simulink model "dspace_2019"  (R2019b)
settings: Solver=FixedStepDiscrete  StartTime=0.0  StopTime=Inf  FixedStep=1e-3  RelTol=1e-3
PostLoadFcn:
  | , if any(exist('dsrtsu_mdlpostloadfcn', 'file') ~= 0), dsrtsu_mdlpostloadfcn('Execute', bdroot); end,
undefined symbols (not defined in the file): ami, amk1_setpoints_1, amk2_setpoints_1, amk3_setpoints_1, amk4_setpoints_1, as, digital, ebs, indicator, mcu_set_dbu_indicator_points, mcu_set_ecu_indicator_points, res_ntm_node_control
libraries: rtican x63, simulink x5, rti1401lib_dio_type3 x4, simulink_extras x1
(part 11 of 16)

== system dspace_2019/CAN RX/ebs_status ==
  clock_time : Clock
  ebs_status1 : rtican/RTICAN Receive (RX)   Reserved1=[]  Reserved2=[]  Reserved3=[]  Reserved4=[]  SfcnMessage=[]  Msg_Struct=[]  BoardTypeNo=[]  BoardNo=[]  ChannelNo=[]  Parameters=[]  DialogFcn=[]  UnitName=[]  Revision=[]  UnitValues=[]  DSProperties=struct('RTI',struct('Version',uint32(5),'BlockType',struct('isSLSource',uint8(1),'isSLSink',uint8(1),'isHWSource',uint8(0),'isHWSink',uint8(0),'isSetup',uint8(0),'isInline',uint8(1),'isNonInline',uint8(0),'isInterrupt',uint8(0),'isChannelwise',uint8(0)),'IOBoardType','RTICAN','UnitType','MESSAGE','Identifier','RX','DialogType','MSVC','BlockSet','RTICAN','SlaveProcessor','CAN'))  RTIBlockInterface=struct('OutputPortsWidth',int32([1 1 1 1 1 1 1]),'OutputPortsActive',[1 1 1 1 1 1 1],'OutputPortsName',{{'SC_TSMS_status','RES_open','ebs_pressure_1','ebs_pressure_2',['RX status'],['RX time'],['RX delta time']}},'OutputPortsDataType',{{'SS_DOUBLE','SS_DOUBLE','SS_DOUBLE','SS_DOUBLE','SS_DOUBLE','SS_DOUBLE','SS_DOUBLE'}},'OutputPortsLabel',{{'SC_TSMS_status','RES_open','ebs_pressure_1','ebs_pressure_2','','',''}},'OutputPortsLabelMode','ON','InputPortsWidth',int32(0),'InputPortsActive',0,'DialogFcn','rtican_message_interface_gui','BlockDisplay',{{'','center'}},'IconTransparency','on','ParameterTunableNames',{{}},'InitLevel',3,'BlockName',struct('Token',{{'ebs_status'}}),'SampleTime',{{-1}},'TriggerPort',{{'none'}},'EnablePort',{{'none'}})  RTIBlockParameters=struct('BoardTypeNo',{{1,'OFF',[]}},'BoardNo',{{1,'ON',[1 16]}},'ChannelNo',{{2,'ON',[1 2]}},'Parameters',{{struct('DataFileSupport',struct('DataFileSelectedMaster',1,'DataFileSelectedLocal',1,'DataFileName','c:\users\oscar\documents\github\sw_infrastructure\kthfspe_python\databases\can1.dbc|','DataFileDate',{{{['10-Jul-2022 16:14:04']}}},'SelectedFile','c:\users\oscar\documents\github\sw_infrastructure\kthfspe_python\databases\can1.dbc'),'Options',struct('StatusSelected',1,'TimeSelected',1,'DeltaTimeSelected',1,'BytePortSelected',0,'MessageLengthSelected',0,'TriggerPort',struct('Selected',0,'TriggerType',0),'UserCoding',struct('Selected',0,'InterfaceFile','UserDecodingFile','FcnName','UserDecodeFcn','InportSelected',0,'InportWidth',1,'OutportSelected',0,'OutportWidth',1),'EnablePortSelected',0,'SignalOnPortnameSelected',1,'UseRXService',0),'Message',struct('MsgOnBlocknameSelected',1,'MsgName','ebs_status','MsgIdFormat',0,'MsgId',80,'MsgLength',4,'NumSignals',4,'SampleTime',-1,'Signal',struct('SgnName',{'SC_TSMS_status','RES_open','ebs_pressure_1','ebs_pressure_2'},'SgnStartBit',{0,1,8,20},'SgnLength',{1,1,12,12},'SgnType',{0,0,0,0},'ModeValue',{-1,-1,-1,-1},'DataType',{0,0,0,0},'ByteLayout',{0,0,0,0},'Factor',{1,1,1,1},'Offset',{0,0,0,0},'SgnComment',{{''},{''},{''},{''}},'SgnUnit',{'','','',''},'Min',{0,0,0,0},'Max',{0,0,0,0},'SLDataType',{'SS_DOUBLE','SS_DOUBLE','SS_DOUBLE','SS_DOUBLE'}),'MsgIdNumFormat',0,'MsgComment',{{''}}),'Version',1.2,'general',struct('isFromLib',0)),'OFF',[]}},'GroupId',{{struct('Group',{{'RTICAN'}},'No',1,'Behavior',{{'NAMECHANGE'}},'BlockType',{{'SINK'}},'NameChangeFlag',0),'OFF',[]}},'SFcnRTICANMessage',{{struct('MsgType','RX','SFcnPortType','Scalar','MsgName','ebs_status','MsgIdFormat','STD','MsgId',80,'MsgLength',4,'NumSignals',4,'SampleTime',-1,'Signal',struct('SgnName',{'SC_TSMS_status','RES_open','ebs_pressure_1','ebs_pressure_2'},'SgnStartBit',{0,1,8,20},'SgnLength',{1,1,12,12},'SgnType',{'standard','standard','standard','standard'},'ModeValue',{-1,-1,-1,-1},'DataType',{['unsigned int'],['unsigned int'],['unsigned int'],['unsigned int']},'ByteLayout',{['little endian'],['little endian'],['little endian'],['little endian']},'Factor',{1,1,1,1},'Offset',{0,0,0,0},'SLDataType',{'SS_DOUBLE','SS_DOUBLE','SS_DOUBLE','SS_DOUBLE'}),'StatusSelected','yes','TimeSelected','yes','DeltaTimeSelected','yes','BytePortSelected','no','MessageLengthSelected','no','TriggerPort',struct('Selected','no','TriggerType',0),'UserCoding',struct('Selected','no','InterfaceFile','UserDecodingFile','FcnName','UserDecodeFcn','InportSelected','no','InportWidth',1,'OutportSelected','no','OutportWidth',1),'EnablePortSelected','no','UseRXService','no','BoardType','DS1','BoardNo',1,'ControllerNo',1),'OFF',[]}},'TLCFileName',{{'rtican_rx_message','OFF',[]}})  RTISFcnParameters=struct('SFcnRTICANMessage','struct','TLCFileName','char')  RTIBlockParaDefault=struct('BoardTypeNo',4302,'BoardNo',1,'ChannelNo',1,'Parameters',struct('DataFileSupport',struct('DataFileSelectedMaster',0,'DataFileSelectedLocal',0,'DataFileName','','DataFileDate','','SelectedFile',['<no file selected>']),'Options',struct('StatusSelected',1,'TimeSelected',1,'DeltaTimeSelected',1,'BytePortSelected',0,'MessageLengthSelected',0,'TriggerPort',struct('Selected',0,'TriggerType','rising'),'UserCoding',struct('Selected',0,'InterfaceFile','UserDecodingFile','FcnName','UserDecodeFcn','InportSelected',0,'InportWidth',1,'OutportSelected',0,'OutportWidth',1),'EnablePortSelected',0,'SignalOnPortnameSelected',1,'UseRXService',0),'Message',struct('MsgOnBlocknameSelected',0,'MsgName',['RX Message'],'MsgIdFormat',0,'MsgId',100,'MsgLength',8,'NumSignals',1,'SampleTime',-1,'Signal',struct('SgnName',['RX signal'],'SgnStartBit',0,'SgnLength',8,'SgnType',0,'ModeValue',-1,'DataType',0,'SLDataType','SS_DOUBLE','ByteLayout',0,'Factor',1,'Offset',0,'Min',0,'Max',255,'SgnComment',{{}},'SgnUnit',''),'MsgIdNumFormat',0,'MsgComment',{{''}}),'Version',1.2,'general',struct('isFromLib',1)),'GroupId',struct('Group',{{'RTICAN'}},'No',1,'Behavior',{{'NAMECHANGE'}},'BlockType',{{'SINK'}},'NameChangeFlag',0),'SFcnRTICANMessage',struct('MsgType','RX','MsgName',['RX Message'],'MsgIdFormat','STD','MsgId',100,'MsgLength',8,'NumSignals',1,'SampleTime',-1,'Signal',struct('SgnName',['RX signal'],'SgnStartBit',0,'SgnLength',8,'SgnType','standard','ModeValue',-1,'DataType',['unsigned int'],'ByteLayout',['little endian'],'SLDataType','SS_DOUBLE','Factor',1,'Offset',0),'StatusSelected','yes','TimeSelected','yes','DeltaTimeSelected','yes','BytePortSelected','no','MessageLengthSelected','no','EnablePortSelected','no','UserCoding',struct('Selected','no','InterfaceFile','UserDecodingFile','FcnName','UserDecodeFcn','InportSelected','no','InportWidth',1,'OutportSelected','no','OutportWidth',1),'TriggerPort',struct('Selected','no','TriggerType','rising'),'UseRXService','no','BoardType','DS4302','BoardNo',1,'ControllerNo',1,'SFcnPortType','Scalar'),'TLCFileName','rtican_rx_message')
      settings: AttributesFormatString=Group Id: RTICAN1\n  SourceProductName=dSPACE RTI CAN Blockset
  sub_time : Sum  Inputs=+-
  SC_TSMS_status_bus : Outport  PortName=signals  Element=SC_TSMS_status
  RES_open_bus : Outport  PortName=signals  Element=RES_open
  ebs_pressure_1_bus : Outport  PortName=signals  Element=ebs_pressure_1
  ebs_pressure_2_bus : Outport  PortName=signals  Element=ebs_pressure_2
  status : Outport  Port=2
  time : Outport  Port=3
  delta : Outport  Port=4
  wires:
  clock_time/1 -> sub_time/1
  sub_time/1 -> time/1
  ebs_status1/5 -> status/1
  ebs_status1/6 -> sub_time/2
  ebs_status1/7 -> delta/1
  ebs_status1/1 -> SC_TSMS_status_bus/1  "SC_TSMS_status"
  ebs_status1/2 -> RES_open_bus/1  "RES_open"
  ebs_status1/3 -> ebs_pressure_1_bus/1  "ebs_pressure_1"
  ebs_status1/4 -> ebs_pressure_2_bus/1  "ebs_pressure_2"

== system dspace_2019/CAN RX/ecu_status ==
  clock_time : Clock
  ecu_status1 : rtican/RTICAN Receive (RX)   Reserved1=[]  Reserved2=[]  Reserved3=[]  Reserved4=[]  SfcnMessage=[]  Msg_Struct=[]  BoardTypeNo=[]  BoardNo=[]  ChannelNo=[]  Parameters=[]  DialogFcn=[]  UnitName=[]  Revision=[]  UnitValues=[]  DSProperties=struct('RTI',struct('Version',uint32(5),'BlockType',struct('isSLSource',uint8(1),'isSLSink',uint8(1),'isHWSource',uint8(0),'isHWSink',uint8(0),'isSetup',uint8(0),'isInline',uint8(1),'isNonInline',uint8(0),'isInterrupt',uint8(0),'isChannelwise',uint8(0)),'IOBoardType','RTICAN','UnitType','MESSAGE','Identifier','RX','DialogType','MSVC','BlockSet','RTICAN','SlaveProcessor','CAN'))  RTIBlockInterface=struct('OutputPortsWidth',int32([1 1 1 1 1 1]),'OutputPortsActive',[1 1 1 1 1 1],'OutputPortsName',{{'rst_button','close_airs','ts_off',['RX status'],['RX time'],['RX delta time']}},'OutputPortsDataType',{{'SS_DOUBLE','SS_DOUBLE','SS_DOUBLE','SS_DOUBLE','SS_DOUBLE','SS_DOUBLE'}},'OutputPortsLabel',{{'rst_button','close_airs','ts_off','','',''}},'OutputPortsLabelMode','ON','InputPortsWidth',int32(0),'InputPortsActive',0,'DialogFcn','rtican_message_interface_gui','BlockDisplay',{{'','center'}},'IconTransparency','on','ParameterTunableNames',{{}},'InitLevel',3,'BlockName',struct('Token',{{'ecu_status'}}),'SampleTime',{{-1}},'TriggerPort',{{'none'}},'EnablePort',{{'none'}})  RTIBlockParameters=struct('BoardTypeNo',{{1,'OFF',[]}},'BoardNo',{{1,'ON',[1 16]}},'ChannelNo',{{2,'ON',[1 2]}},'Parameters',{{struct('DataFileSupport',struct('DataFileSelectedMaster',1,'DataFileSelectedLocal',1,'DataFileName','c:\users\oscar\documents\github\sw_infrastructure\kthfspe_python\databases\can1.dbc|','DataFileDate',{{{['10-Jul-2022 16:14:04']}}},'SelectedFile','c:\users\oscar\documents\github\sw_infrastructure\kthfspe_python\databases\can1.dbc'),'Options',struct('StatusSelected',1,'TimeSelected',1,'DeltaTimeSelected',1,'BytePortSelected',0,'MessageLengthSelected',0,'TriggerPort',struct('Selected',0,'TriggerType',0),'UserCoding',struct('Selected',0,'InterfaceFile','UserDecodingFile','FcnName','UserDecodeFcn','InportSelected',0,'InportWidth',1,'OutportSelected',0,'OutportWidth',1),'EnablePortSelected',0,'SignalOnPortnameSelected',1,'UseRXService',0),'Message',struct('MsgOnBlocknameSelected',1,'MsgName','ecu_status','MsgIdFormat',0,'MsgId',72,'MsgLength',8,'NumSignals',3,'SampleTime',-1,'Signal',struct('SgnName',{'rst_button','close_airs','ts_off'},'SgnStartBit',{0,8,16},'SgnLength',{8,8,8},'SgnType',{0,0,0},'ModeValue',{-1,-1,-1},'DataType',{0,0,0},'ByteLayout',{0,0,0},'Factor',{1,1,1},'Offset',{0,0,0},'SgnComment',{{''},{''},{''}},'SgnUnit',{'','',''},'Min',{0,0,0},'Max',{0,0,0},'SLDataType',{'SS_DOUBLE','SS_DOUBLE','SS_DOUBLE'}),'MsgIdNumFormat',0,'MsgComment',{{''}}),'Version',1.2,'general',struct('isFromLib',0)),'OFF',[]}},'GroupId',{{struct('Group',{{'RTICAN'}},'No',1,'Behavior',{{'NAMECHANGE'}},'BlockType',{{'SINK'}},'NameChangeFlag',0),'OFF',[]}},'SFcnRTICANMessage',{{struct('MsgType','RX','SFcnPortType','Scalar','MsgName','ecu_status','MsgIdFormat','STD','MsgId',72,'MsgLength',8,'NumSignals',3,'SampleTime',-1,'Signal',struct('SgnName',{'rst_button','close_airs','ts_off'},'SgnStartBit',{0,8,16},'SgnLength',{8,8,8},'SgnType',{'standard','standard','standard'},'ModeValue',{-1,-1,-1},'DataType',{['unsigned int'],['unsigned int'],['unsigned int']},'ByteLayout',{['little endian'],['little endian'],['little endian']},'Factor',{1,1,1},'Offset',{0,0,0},'SLDataType',{'SS_DOUBLE','SS_DOUBLE','SS_DOUBLE'}),'StatusSelected','yes','TimeSelected','yes','DeltaTimeSelected','yes','BytePortSelected','no','MessageLengthSelected','no','TriggerPort',struct('Selected','no','TriggerType',0),'UserCoding',struct('Selected','no','InterfaceFile','UserDecodingFile','FcnName','UserDecodeFcn','InportSelected','no','InportWidth',1,'OutportSelected','no','OutportWidth',1),'EnablePortSelected','no','UseRXService','no','BoardType','DS1','BoardNo',1,'ControllerNo',1),'OFF',[]}},'TLCFileName',{{'rtican_rx_message','OFF',[]}})  RTISFcnParameters=struct('SFcnRTICANMessage','struct','TLCFileName','char')  RTIBlockParaDefault=struct('BoardTypeNo',4302,'BoardNo',1,'ChannelNo',1,'Parameters',struct('DataFileSupport',struct('DataFileSelectedMaster',0,'DataFileSelectedLocal',0,'DataFileName','','DataFileDate','','SelectedFile',['<no file selected>']),'Options',struct('StatusSelected',1,'TimeSelected',1,'DeltaTimeSelected',1,'BytePortSelected',0,'MessageLengthSelected',0,'TriggerPort',struct('Selected',0,'TriggerType','rising'),'UserCoding',struct('Selected',0,'InterfaceFile','UserDecodingFile','FcnName','UserDecodeFcn','InportSelected',0,'InportWidth',1,'OutportSelected',0,'OutportWidth',1),'EnablePortSelected',0,'SignalOnPortnameSelected',1,'UseRXService',0),'Message',struct('MsgOnBlocknameSelected',0,'MsgName',['RX Message'],'MsgIdFormat',0,'MsgId',100,'MsgLength',8,'NumSignals',1,'SampleTime',-1,'Signal',struct('SgnName',['RX signal'],'SgnStartBit',0,'SgnLength',8,'SgnType',0,'ModeValue',-1,'DataType',0,'SLDataType','SS_DOUBLE','ByteLayout',0,'Factor',1,'Offset',0,'Min',0,'Max',255,'SgnComment',{{}},'SgnUnit',''),'MsgIdNumFormat',0,'MsgComment',{{''}}),'Version',1.2,'general',struct('isFromLib',1)),'GroupId',struct('Group',{{'RTICAN'}},'No',1,'Behavior',{{'NAMECHANGE'}},'BlockType',{{'SINK'}},'NameChangeFlag',0),'SFcnRTICANMessage',struct('MsgType','RX','MsgName',['RX Message'],'MsgIdFormat','STD','MsgId',100,'MsgLength',8,'NumSignals',1,'SampleTime',-1,'Signal',struct('SgnName',['RX signal'],'SgnStartBit',0,'SgnLength',8,'SgnType','standard','ModeValue',-1,'DataType',['unsigned int'],'ByteLayout',['little endian'],'SLDataType','SS_DOUBLE','Factor',1,'Offset',0),'StatusSelected','yes','TimeSelected','yes','DeltaTimeSelected','yes','BytePortSelected','no','MessageLengthSelected','no','EnablePortSelected','no','UserCoding',struct('Selected','no','InterfaceFile','UserDecodingFile','FcnName','UserDecodeFcn','InportSelected','no','InportWidth',1,'OutportSelected','no','OutportWidth',1),'TriggerPort',struct('Selected','no','TriggerType','rising'),'UseRXService','no','BoardType','DS4302','BoardNo',1,'ControllerNo',1,'SFcnPortType','Scalar'),'TLCFileName','rtican_rx_message')
      settings: AttributesFormatString=Group Id: RTICAN1\n  SourceProductName=dSPACE RTI CAN Blockset
  sub_time : Sum  Inputs=+-
  rst_button_bus : Outport  PortName=signals  Element=rst_button
  close_airs_bus : Outport  PortName=signals  Element=close_airs
  ts_off_bus : Outport  PortName=signals  Element=ts_off
  status : Outport  Port=2
  time : Outport  Port=3
  delta : Outport  Port=4
  wires:
  clock_time/1 -> sub_time/1
  sub_time/1 -> time/1
  ecu_status1/4 -> status/1
  ecu_status1/5 -> sub_time/2
  ecu_status1/6 -> delta/1
  ecu_status1/1 -> rst_button_bus/1  "rst_button"
  ecu_status1/2 -> close_airs_bus/1  "close_airs"
  ecu_status1/3 -> ts_off_bus/1  "ts_off"

== system dspace_2019/CAN RX/fault ==
  clock_time : Clock
  fault1 : rtican/RTICAN Receive (RX)   Reserved1=[]  Reserved2=[]  Reserved3=[]  Reserved4=[]  SfcnMessage=[]  Msg_Struct=[]  BoardTypeNo=[]  BoardNo=[]  ChannelNo=[]  Parameters=[]  DialogFcn=[]  UnitName=[]  Revision=[]  UnitValues=[]  DSProperties=struct('RTI',struct('Version',uint32(5),'BlockType',struct('isSLSource',uint8(1),'isSLSink',uint8(1),'isHWSource',uint8(0),'isHWSink',uint8(0),'isSetup',uint8(0),'isInline',uint8(1),'isNonInline',uint8(0),'isInterrupt',uint8(0),'isChannelwise',uint8(0)),'IOBoardType','RTICAN','UnitType','MESSAGE','Identifier','RX','DialogType','MSVC','BlockSet','RTICAN','SlaveProcessor','CAN'))  RTIBlockInterface=struct('OutputPortsWidth',int32([1 1 1 1 1 1 1 1 1 1 1 1 1 1]),'OutputPortsActive',ones(1,14),'OutputPortsName',{{'unit_id','sc_open','ts_off_watchdog_triggered','apps_discrepancy','bpps_discrepancy','brake_pressure_discrepancy','steering_angle_discrepancy','apps_out_of_range','bpps_out_of_range','brake_pressure_out_of_range','steering_angle_out_of_range',['RX status'],['RX time'],['RX delta time']}},'OutputPortsDataType',{{'SS_DOUBLE','SS_DOUBLE','SS_DOUBLE','SS_DOUBLE','SS_DOUBLE','SS_DOUBLE','SS_DOUBLE','SS_DOUBLE','SS_DOUBLE','SS_DOUBLE','SS_DOUBLE','SS_DOUBLE','SS_DOUBLE','SS_DOUBLE'}},'OutputPortsLabel',{{'unit_id','sc_open','ts_off_watchdog_triggered','apps_discrepancy','bpps_discrepancy','brake_pressure_discrepancy','steering_angle_discrepancy','apps_out_of_range','bpps_out_of_range','brake_pressure_out_of_range','steering_angle_out_of_range','','',''}},'OutputPortsLabelMode','ON','InputPortsWidth',int32(0),'InputPortsActive',0,'DialogFcn','rtican_message_interface_gui','BlockDisplay',{{'','center'}},'IconTransparency','on','ParameterTunableNames',{{}},'InitLevel',3,'BlockName',struct('Token',{{'fault'}}),'SampleTime',{{-1}},'TriggerPort',{{'none'}},'EnablePort',{{'none'}})  RTIBlockParameters=struct('BoardTypeNo',{{1,'OFF',[]}},'BoardNo',{{1,'ON',[1 16]}},'ChannelNo',{{2,'ON',[1 2]}},'Parameters',{{struct('DataFileSupport',struct('DataFileSelectedMaster',1,'DataFileSelectedLocal',1,'DataFileName','c:\users\oscar\documents\github\sw_infrastructure\kthfspe_python\databases\can1.dbc|','DataFileDate',{{{['10-Jul-2022 16:14:04']}}},'SelectedFile','c:\users\oscar\documents\github\sw_infrastructure\kthfspe_python\databases\can1.dbc'),'Options',struct('StatusSelected',1,'TimeSelected',1,'DeltaTimeSelected',1,'BytePortSelected',0,'MessageLengthSelected',0,'TriggerPort',struct('Selected',0,'TriggerType',0),'UserCoding',struct('Selected',0,'InterfaceFile','UserDecodingFile','FcnName','UserDecodeFcn','InportSelected',0,'InportWidth',1,'OutportSelected',0,'OutportWidth',1),'EnablePortSelected',0,'SignalOnPortnameSelected',1,'UseRXService',0),'Message',struct('MsgOnBlocknameSelected',1,'MsgName','fault','MsgIdFormat',0,'MsgId',255,'MsgLength',8,'NumSignals',11,'SampleTime',-1,'Signal',struct('SgnName',{'unit_id','sc_open','ts_off_watchdog_triggered','apps_discrepancy','bpps_discrepancy','brake_pressure_discrepancy','steering_angle_discrepancy','apps_out_of_range','bpps_out_of_range','brake_pressure_out_of_range','steering_angle_out_of_range'},'SgnStartBit',{0,8,8,8,9,10,11,12,13,14,15},'SgnLength',{8,1,1,1,1,1,1,1,1,1,1},'SgnType',{1,2,2,2,2,2,2,2,2,2,2},'ModeValue',{-1,0,3,4,4,4,0,4,4,4,4},'DataType',{0,0,0,0,0,0,0,0,0,0,0},'ByteLayout',{0,0,0,0,0,0,0,0,0,0,0},'Factor',{1,1,1,1,1,1,1,1,1,1,1},'Offset',{0,0,0,0,0,0,0,0,0,0,0},'SgnComment',{{''},{''},{''},{''},{''},{''},{''},{''},{''},{''},{''}},'SgnUnit',{'','','','','','','','','','',''},'Min',{0,0,0,0,0,0,0,0,0,0,0},'Max',{0,0,0,0,0,0,0,0,0,0,0},'SLDataType',{'SS_DOUBLE','SS_DOUBLE','SS_DOUBLE','SS_DOUBLE','SS_DOUBLE','SS_DOUBLE','SS_DOUBLE','SS_DOUBLE','SS_DOUBLE','SS_DOUBLE','SS_DOUBLE'}),'MsgIdNumFormat',0,'MsgComment',{{''}}),'Version',1.2,'general',struct('isFromLib',0)),'OFF',[]}},'GroupId',{{struct('Group',{{'RTICAN'}},'No',1,'Behavior',{{'NAMECHANGE'}},'BlockType',{{'SINK'}},'NameChangeFlag',0),'OFF',[]}},'SFcnRTICANMessage',{{struct('MsgType','RX','SFcnPortType','Scalar','MsgName','fault','MsgIdFormat','STD','MsgId',255,'MsgLength',8,'NumSignals',11,'SampleTime',-1,'Signal',struct('SgnName',{'unit_id','sc_open','ts_off_watchdog_triggered','apps_discrepancy','bpps_discrepancy','brake_pressure_discrepancy','steering_angle_discrepancy','apps_out_of_range','bpps_out_of_range','brake_pressure_out_of_range','steering_angle_out_of_range'},'SgnStartBit',{0,8,8,8,9,10,11,12,13,14,15},'SgnLength',{8,1,1,1,1,1,1,1,1,1,1},'SgnType',{'mode','mode-dependent','mode-dependent','mode-dependent','mode-dependent','mode-dependent','mode-dependent','mode-dependent','mode-dependent','mode-dependent','mode-dependent'},'ModeValue',{-1,0,3,4,4,4,0,4,4,4,4},'DataType',{['unsigned int'],['unsigned int'],['unsigned int'],['unsigned int'],['unsigned int'],['unsigned int'],['unsigned int'],['unsigned int'],['unsigned int'],['unsigned int'],['unsigned int']},'ByteLayout',{['little endian'],['little endian'],['little endian'],['little endian'],['little endian'],['little endian'],['little endian'],['little endian'],['little endian'],['little endian'],['little endian']},'Factor',{1,1,1,1,1,1,1,1,1,1,1},'Offset',{0,0,0,0,0,0,0,0,0,0,0},'SLDataType',{'SS_DOUBLE','SS_DOUBLE','SS_DOUBLE','SS_DOUBLE','SS_DOUBLE','SS_DOUBLE','SS_DOUBLE','SS_DOUBLE','SS_DOUBLE','SS_DOUBLE','SS_DOUBLE'}),'StatusSelected','yes','TimeSelected','yes','DeltaTimeSelected','yes','BytePortSelected','no','MessageLengthSelected','no','TriggerPort',struct('Selected','no','TriggerType',0),'UserCoding',struct('Selected','no','InterfaceFile','UserDecodingFile','FcnName','UserDecodeFcn','InportSelected','no','InportWidth',1,'OutportSelected','no','OutportWidth',1),'EnablePortSelected','no','UseRXService','no','BoardType','DS1','BoardNo',1,'ControllerNo',1),'OFF',[]}},'TLCFileName',{{'rtican_rx_message','OFF',[]}})  RTISFcnParameters=struct('SFcnRTICANMessage','struct','TLCFileName','char')  RTIBlockParaDefault=struct('BoardTypeNo',4302,'BoardNo',1,'ChannelNo',1,'Parameters',struct('DataFileSupport',struct('DataFileSelectedMaster',0,'DataFileSelectedLocal',0,'DataFileName','','DataFileDate','','SelectedFile',['<no file selected>']),'Options',struct('StatusSelected',1,'TimeSelected',1,'DeltaTimeSelected',1,'BytePortSelected',0,'MessageLengthSelected',0,'TriggerPort',struct('Selected',0,'TriggerType','rising'),'UserCoding',struct('Selected',0,'InterfaceFile','UserDecodingFile','FcnName','UserDecodeFcn','InportSelected',0,'InportWidth',1,'OutportSelected',0,'OutportWidth',1),'EnablePortSelected',0,'SignalOnPortnameSelected',1,'UseRXService',0),'Message',struct('MsgOnBlocknameSelected',0,'MsgName',['RX Message'],'MsgIdFormat',0,'MsgId',100,'MsgLength',8,'NumSignals',1,'SampleTime',-1,'Signal',struct('SgnName',['RX signal'],'SgnStartBit',0,'SgnLength',8,'SgnType',0,'ModeValue',-1,'DataType',0,'SLDataType','SS_DOUBLE','ByteLayout',0,'Factor',1,'Offset',0,'Min',0,'Max',255,'SgnComment',{{}},'SgnUnit',''),'MsgIdNumFormat',0,'MsgComment',{{''}}),'Version',1.2,'general',struct('isFromLib',1)),'GroupId',struct('Group',{{'RTICAN'}},'No',1,'Behavior',{{'NAMECHANGE'}},'BlockType',{{'SINK'}},'NameChangeFlag',0),'SFcnRTICANMessage',struct('MsgType','RX','MsgName',['RX Message'],'MsgIdFormat','STD','MsgId',100,'MsgLength',8,'NumSignals',1,'SampleTime',-1,'Signal',struct('SgnName',['RX signal'],'SgnStartBit',0,'SgnLength',8,'SgnType','standard','ModeValue',-1,'DataType',['unsigned int'],'ByteLayout',['little endian'],'SLDataType','SS_DOUBLE','Factor',1,'Offset',0),'StatusSelected','yes','TimeSelected','yes','DeltaTimeSelected','yes','BytePortSelected','no','MessageLengthSelected','no','EnablePortSelected','no','UserCoding',struct('Selected','no','InterfaceFile','UserDecodingFile','FcnName','UserDecodeFcn','InportSelected','no','InportWidth',1,'OutportSelected','no','OutportWidth',1),'TriggerPort',struct('Selected','no','TriggerType','rising'),'UseRXService','no','BoardType','DS4302','BoardNo',1,'ControllerNo',1,'SFcnPortType','Scalar'),'TLCFileName','rtican_rx_message')
      settings: AttributesFormatString=Group Id: RTICAN1\n  SourceProductName=dSPACE RTI CAN Blockset
  sub_time : Sum  Inputs=+-
  unit_id_bus : Outport  PortName=signals  Element=unit_id
  apps_discrepancy_bus : Outport  PortName=signals  Element=apps_discrepancy
  sc_open_bus : Outport  PortName=signals  Element=sc_open
  ts_off_watchdog_triggered_bus : Outport  PortName=signals  Element=ts_off_watchdog_triggered
  bpps_discrepancy_bus : Outport  PortName=signals  Element=bpps_discrepancy
  brake_pressure_discrepancy_bus : Outport  PortName=signals  Element=brake_pressure_discrepancy
  steering_angle_discrepancy_bus : Outport  PortName=signals  Element=steering_angle_discrepancy
  apps_out_of_range_bus : Outport  PortName=signals  Element=apps_out_of_range
  bpps_out_of_range_bus : Outport  PortName=signals  Element=bpps_out_of_range
  brake_pressure_out_of_range_bus : Outport  PortName=signals  Element=brake_pressure_out_of_range
  steering_angle_out_of_range_bus : Outport  PortName=signals  Element=steering_angle_out_of_range
  status : Outport  Port=2
  time : Outport  Port=3
  delta : Outport  Port=4
  wires:
  clock_time/1 -> sub_time/1
  sub_time/1 -> time/1
  fault1/12 -> status/1
  fault1/13 -> sub_time/2
  fault1/14 -> delta/1
  fault1/1 -> unit_id_bus/1  "unit_id"
  fault1/2 -> apps_discrepancy_bus/1  "sc_open"
  fault1/3 -> sc_open_bus/1  "ts_off_watchdog_triggered"
  fault1/4 -> ts_off_watchdog_triggered_bus/1  "apps_discrepancy"
  fault1/5 -> bpps_discrepancy_bus/1  "bpps_discrepancy"
  fault1/6 -> brake_pressure_discrepancy_bus/1  "brake_pressure_discrepancy"
  fault1/7 -> steering_angle_discrepancy_bus/1  "steering_angle_discrepancy"
  fault1/8 -> apps_out_of_range_bus/1  "apps_out_of_range"
  fault1/9 -> bpps_out_of_range_bus/1  "bpps_out_of_range"
  fault1/10 -> brake_pressure_out_of_range_bus/1  "brake_pressure_out_of_range"
  fault1/11 -> steering_angle_out_of_range_bus/1  "steering_angle_out_of_range"

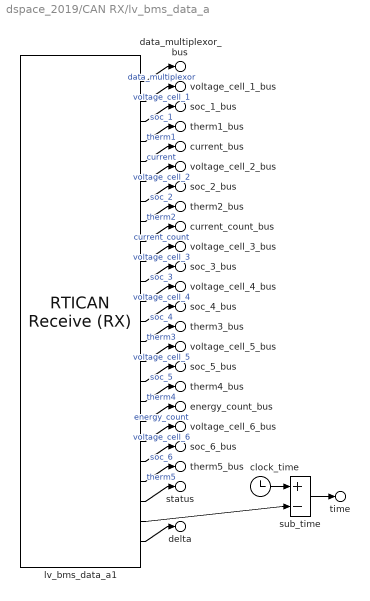
== system dspace_2019/CAN RX/lv_bms_data_a ==
  clock_time : Clock
  lv_bms_data_a1 : rtican/RTICAN Receive (RX)   Reserved1=[]  Reserved2=[]  Reserved3=[]  Reserved4=[]  SfcnMessage=[]  Msg_Struct=[]  BoardTypeNo=[]  BoardNo=[]  ChannelNo=[]  Parameters=[]  DialogFcn=[]  UnitName=[]  Revision=[]  UnitValues=[]  DSProperties=struct('RTI',struct('Version',uint32(5),'BlockType',struct('isSLSource',uint8(1),'isSLSink',uint8(1),'isHWSource',uint8(0),'isHWSink',uint8(0),'isSetup',uint8(0),'isInline',uint8(1),'isNonInline',uint8(0),'isInterrupt',uint8(0),'isChannelwise',uint8(0)),'IOBoardType','RTICAN','UnitType','MESSAGE','Identifier','RX','DialogType','MSVC','BlockSet','RTICAN','SlaveProcessor','CAN'))  RTIBlockInterface=struct('OutputPortsWidth',int32([1 1 1 1 1 1 1 1 1 1 1 1 1 1 1 1 1 1 1 1 1 1 1 1]),'OutputPortsActive',ones(1,24),'OutputPortsName',{{'data_multiplexor','voltage_cell_1','soc_1','therm1','current','voltage_cell_2','soc_2','therm2','current_count','voltage_cell_3','soc_3','voltage_cell_4','soc_4','therm3','voltage_cell_5','soc_5','therm4','energy_count','voltage_cell_6','soc_6','therm5',['RX status'],['RX time'],['RX delta time']}},'OutputPortsDataType',{{'SS_DOUBLE','SS_DOUBLE','SS_DOUBLE','SS_DOUBLE','SS_DOUBLE','SS_DOUBLE','SS_DOUBLE','SS_DOUBLE','SS_DOUBLE','SS_DOUBLE','SS_DOUBLE','SS_DOUBLE','SS_DOUBLE','SS_DOUBLE','SS_DOUBLE','SS_DOUBLE','SS_DOUBLE','SS_DOUBLE','SS_DOUBLE','SS_DOUBLE','SS_DOUBLE','SS_DOUBLE','SS_DOUBLE','SS_DOUBLE'}},'OutputPortsLabel',{{'data_multiplexor','voltage_cell_1','soc_1','therm1','current','voltage_cell_2','soc_2','therm2','current_count','voltage_cell_3','soc_3','voltage_cell_4','soc_4','therm3','voltage_cell_5','soc_5','therm4','energy_count','voltage_cell_6','soc_6','therm5','','',''}},'OutputPortsLabelMode','ON','InputPortsWidth',int32(0),'InputPortsActive',0,'DialogFcn','rtican_message_interface_gui','BlockDisplay',{{'','center'}},'IconTransparency','on','ParameterTunableNames',{{}},'InitLevel',3,'BlockName',struct('Token',{{'lv_bms_data_a'}}),'SampleTime',{{-1}},'TriggerPort',{{'none'}},'EnablePort',{{'none'}})  RTIBlockParameters=struct('BoardTypeNo',{{1,'OFF',[]}},'BoardNo',{{1,'ON',[1 16]}},'ChannelNo',{{2,'ON',[1 2]}},'Parameters',{{struct('DataFileSupport',struct('DataFileSelectedMaster',1,'DataFileSelectedLocal',1,'DataFileName','c:\users\oscar\documents\github\sw_infrastructure\kthfspe_python\databases\can1.dbc|','DataFileDate',{{{['10-Jul-2022 15:50:24']}}},'SelectedFile','c:\users\oscar\documents\github\sw_infrastructure\kthfspe_python\databases\can1.dbc'),'Options',struct('StatusSelected',1,'TimeSelected',1,'DeltaTimeSelected',1,'BytePortSelected',0,'MessageLengthSelected',0,'TriggerPort',struct('Selected',0,'TriggerType',0),'UserCoding',struct('Selected',0,'InterfaceFile','UserDecodingFile','FcnName','UserDecodeFcn','InportSelected',0,'InportWidth',1,'OutportSelected',0,'OutportWidth',1),'EnablePortSelected',0,'SignalOnPortnameSelected',1,'UseRXService',0),'Message',struct('MsgOnBlocknameSelected',1,'MsgName','lv_bms_data_a','MsgIdFormat',0,'MsgId',100,'MsgLength',8,'NumSignals',21,'SampleTime',-1,'Signal',struct('SgnName',{'data_multiplexor','voltage_cell_1','soc_1','therm1','current','voltage_cell_2','soc_2','therm2','current_count','voltage_cell_3','soc_3','voltage_cell_4','soc_4','therm3','voltage_cell_5','soc_5','therm4','energy_count','voltage_cell_6','soc_6','therm5'},'SgnStartBit',{0,4,4,4,4,12,12,16,16,20,20,28,28,28,36,36,40,40,44,44,52},'SgnLength',{3,8,8,12,12,8,8,12,24,8,8,8,8,12,8,8,12,24,8,8,12},'SgnType',{1,2,2,2,2,2,2,2,2,2,2,2,2,2,2,2,2,2,2,2,2},'ModeValue',{-1,0,1,2,3,0,1,2,3,0,1,0,1,2,0,1,2,3,0,1,2},'DataType',{0,0,0,1,0,0,0,1,0,0,0,0,0,1,0,0,1,0,0,0,1},'ByteLayout',{0,0,0,0,0,0,0,0,0,0,0,0,0,0,0,0,0,0,0,0,0},'Factor',{1,0.007843,0.003922,0.04884,0.004884,0.007843,0.003922,0.04884,0.021243,0.007843,0.003922,0.007843,0.003922,0.04884,0.007843,0.003922,0.04884,0.091345,0.007843,0.003922,0.04884},'Offset',{0,2.5,0,-10,0,2.5,0,-10,0,2.5,0,2.5,0,-10,2.5,0,-10,0,2.5,0,-10},'SgnComment',{{''},{''},{''},{''},{''},{''},{''},{''},{''},{''},{''},{''},{''},{''},{''},{''},{''},{''},{''},{''},{''}},'SgnUnit',{'','V','%','C','A','V','%','C','As','V','%','V','%','C','V','%','C','Ws','V','%','C'},'Min',{0,2.5,0,-10,0,2.5,0,-10,0,2.5,0,2.5,0,-10,2.5,0,-10,0,2.5,0,-10},'Max',{0,4.5,1,190,20,4.5,1,190,356400,4.5,1,4.5,1,190,4.5,1,190,1532520,4.5,1,190},'SLDataType',{'SS_DOUBLE','SS_DOUBLE','SS_DOUBLE','SS_DOUBLE','SS_DOUBLE','SS_DOUBLE','SS_DOUBLE','SS_DOUBLE','SS_DOUBLE','SS_DOUBLE','SS_DOUBLE','SS_DOUBLE','SS_DOUBLE','SS_DOUBLE','SS_DOUBLE','SS_DOUBLE','SS_DOUBLE','SS_DOUBLE','SS_DOUBLE','SS_DOUBLE','SS_DOUBLE'}),'MsgIdNumFormat',0,'MsgComment',{{''}}),'Version',1.2,'general',struct('isFromLib',0)),'OFF',[]}},'GroupId',{{struct('Group',{{'RTICAN'}},'No',1,'Behavior',{{'NAMECHANGE'}},'BlockType',{{'SINK'}},'NameChangeFlag',0),'OFF',[]}},'SFcnRTICANMessage',{{struct('MsgType','RX','SFcnPortType','Scalar','MsgName','lv_bms_data_a','MsgIdFormat','STD','MsgId',100,'MsgLength',8,'NumSignals',21,'SampleTime',-1,'Signal',struct('SgnName',{'data_multiplexor','voltage_cell_1','soc_1','therm1','current','voltage_cell_2','soc_2','therm2','current_count','voltage_cell_3','soc_3','voltage_cell_4','soc_4','therm3','voltage_cell_5','soc_5','therm4','energy_count','voltage_cell_6','soc_6','therm5'},'SgnStartBit',{0,4,4,4,4,12,12,16,16,20,20,28,28,28,36,36,40,40,44,44,52},'SgnLength',{3,8,8,12,12,8,8,12,24,8,8,8,8,12,8,8,12,24,8,8,12},'SgnType',{'mode','mode-dependent','mode-dependent','mode-dependent','mode-dependent','mode-dependent','mode-dependent','mode-dependent','mode-dependent','mode-dependent','mode-dependent','mode-dependent','mode-dependent','mode-dependent','mode-dependent','mode-dependent','mode-dependent','mode-dependent','mode-dependent','mode-dependent','mode-dependent'},'ModeValue',{-1,0,1,2,3,0,1,2,3,0,1,0,1,2,0,1,2,3,0,1,2},'DataType',{['unsigned int'],['unsigned int'],['unsigned int'],['signed int'],['unsigned int'],['unsigned int'],['unsigned int'],['signed int'],['unsigned int'],['unsigned int'],['unsigned int'],['unsigned int'],['unsigned int'],['signed int'],['unsigned int'],['unsigned int'],['signed int'],['unsigned int'],['unsigned int'],['unsigned int'],['signed int']},'ByteLayout',{['little endian'],['little endian'],['little endian'],['little endian'],['little endian'],['little endian'],['little endian'],['little endian'],['little endian'],['little endian'],['little endian'],['little endian'],['little endian'],['little endian'],['little endian'],['little endian'],['little endian'],['little endian'],['little endian'],['little endian'],['little endian']},'Factor',{1,0.007843,0.003922,0.04884,0.004884,0.007843,0.003922,0.04884,0.021243,0.007843,0.003922,0.007843,0.003922,0.04884,0.007843,0.003922,0.04884,0.091345,0.007843,0.003922,0.04884},'Offset',{0,2.5,0,-10,0,2.5,0,-10,0,2.5,0,2.5,0,-10,2.5,0,-10,0,2.5,0,-10},'SLDataType',{'SS_DOUBLE','SS_DOUBLE','SS_DOUBLE','SS_DOUBLE','SS_DOUBLE','SS_DOUBLE','SS_DOUBLE','SS_DOUBLE','SS_DOUBLE','SS_DOUBLE','SS_DOUBLE','SS_DOUBLE','SS_DOUBLE','SS_DOUBLE','SS_DOUBLE','SS_DOUBLE','SS_DOUBLE','SS_DOUBLE','SS_DOUBLE','SS_DOUBLE','SS_DOUBLE'}),'StatusSelected','yes','TimeSelected','yes','DeltaTimeSelected','yes','BytePortSelected','no','MessageLengthSelected','no','TriggerPort',struct('Selected','no','TriggerType',0),'UserCoding',struct('Selected','no','InterfaceFile','UserDecodingFile','FcnName','UserDecodeFcn','InportSelected','no','InportWidth',1,'OutportSelected','no','OutportWidth',1),'EnablePortSelected','no','UseRXService','no','BoardType','DS1','BoardNo',1,'ControllerNo',1),'OFF',[]}},'TLCFileName',{{'rtican_rx_message','OFF',[]}})  RTISFcnParameters=struct('SFcnRTICANMessage','struct','TLCFileName','char')  RTIBlockParaDefault=struct('BoardTypeNo',4302,'BoardNo',1,'ChannelNo',1,'Parameters',struct('DataFileSupport',struct('DataFileSelectedMaster',0,'DataFileSelectedLocal',0,'DataFileName','','DataFileDate','','SelectedFile',['<no file selected>']),'Options',struct('StatusSelected',1,'TimeSelected',1,'DeltaTimeSelected',1,'BytePortSelected',0,'MessageLengthSelected',0,'TriggerPort',struct('Selected',0,'TriggerType','rising'),'UserCoding',struct('Selected',0,'InterfaceFile','UserDecodingFile','FcnName','UserDecodeFcn','InportSelected',0,'InportWidth',1,'OutportSelected',0,'OutportWidth',1),'EnablePortSelected',0,'SignalOnPortnameSelected',1,'UseRXService',0),'Message',struct('MsgOnBlocknameSelected',0,'MsgName',['RX Message'],'MsgIdFormat',0,'MsgId',100,'MsgLength',8,'NumSignals',1,'SampleTime',-1,'Signal',struct('SgnName',['RX signal'],'SgnStartBit',0,'SgnLength',8,'SgnType',0,'ModeValue',-1,'DataType',0,'SLDataType','SS_DOUBLE','ByteLayout',0,'Factor',1,'Offset',0,'Min',0,'Max',255,'SgnComment',{{}},'SgnUnit',''),'MsgIdNumFormat',0,'MsgComment',{{''}}),'Version',1.2,'general',struct('isFromLib',1)),'GroupId',struct('Group',{{'RTICAN'}},'No',1,'Behavior',{{'NAMECHANGE'}},'BlockType',{{'SINK'}},'NameChangeFlag',0),'SFcnRTICANMessage',struct('MsgType','RX','MsgName',['RX Message'],'MsgIdFormat','STD','MsgId',100,'MsgLength',8,'NumSignals',1,'SampleTime',-1,'Signal',struct('SgnName',['RX signal'],'SgnStartBit',0,'SgnLength',8,'SgnType','standard','ModeValue',-1,'DataType',['unsigned int'],'ByteLayout',['little endian'],'SLDataType','SS_DOUBLE','Factor',1,'Offset',0),'StatusSelected','yes','TimeSelected','yes','DeltaTimeSelected','yes','BytePortSelected','no','MessageLengthSelected','no','EnablePortSelected','no','UserCoding',struct('Selected','no','InterfaceFile','UserDecodingFile','FcnName','UserDecodeFcn','InportSelected','no','InportWidth',1,'OutportSelected','no','OutportWidth',1),'TriggerPort',struct('Selected','no','TriggerType','rising'),'UseRXService','no','BoardType','DS4302','BoardNo',1,'ControllerNo',1,'SFcnPortType','Scalar'),'TLCFileName','rtican_rx_message')
      settings: AttributesFormatString=Group Id: RTICAN1\n  SourceProductName=dSPACE RTI CAN Blockset
  sub_time : Sum  Inputs=+-
  data_multiplexor_bus : Outport  PortName=signals  Element=data_multiplexor
  voltage_cell_1_bus : Outport  PortName=signals  Element=voltage_cell_1
  soc_1_bus : Outport  PortName=signals  Element=soc_1
  therm1_bus : Outport  PortName=signals  Element=therm1
  current_bus : Outport  PortName=signals  Element=current
  voltage_cell_2_bus : Outport  PortName=signals  Element=voltage_cell_2
  soc_2_bus : Outport  PortName=signals  Element=soc_2
  therm2_bus : Outport  PortName=signals  Element=therm2
  current_count_bus : Outport  PortName=signals  Element=current_count
  voltage_cell_3_bus : Outport  PortName=signals  Element=voltage_cell_3
  soc_3_bus : Outport  PortName=signals  Element=soc_3
  voltage_cell_4_bus : Outport  PortName=signals  Element=voltage_cell_4
  soc_4_bus : Outport  PortName=signals  Element=soc_4
  therm3_bus : Outport  PortName=signals  Element=therm3
  voltage_cell_5_bus : Outport  PortName=signals  Element=voltage_cell_5
  soc_5_bus : Outport  PortName=signals  Element=soc_5
  therm4_bus : Outport  PortName=signals  Element=therm4
  energy_count_bus : Outport  PortName=signals  Element=energy_count
  voltage_cell_6_bus : Outport  PortName=signals  Element=voltage_cell_6
  soc_6_bus : Outport  PortName=signals  Element=soc_6
  therm5_bus : Outport  PortName=signals  Element=therm5
  status : Outport  Port=2
  time : Outport  Port=3
  delta : Outport  Port=4
  wires:
  clock_time/1 -> sub_time/1
  sub_time/1 -> time/1
  lv_bms_data_a1/22 -> status/1
  lv_bms_data_a1/23 -> sub_time/2
  lv_bms_data_a1/24 -> delta/1
  lv_bms_data_a1/1 -> data_multiplexor_bus/1  "data_multiplexor"
  lv_bms_data_a1/2 -> voltage_cell_1_bus/1  "voltage_cell_1"
  lv_bms_data_a1/3 -> soc_1_bus/1  "soc_1"
  lv_bms_data_a1/4 -> therm1_bus/1  "therm1"
  lv_bms_data_a1/5 -> current_bus/1  "current"
  lv_bms_data_a1/6 -> voltage_cell_2_bus/1  "voltage_cell_2"
  lv_bms_data_a1/7 -> soc_2_bus/1  "soc_2"
  lv_bms_data_a1/8 -> therm2_bus/1  "therm2"
  lv_bms_data_a1/9 -> current_count_bus/1  "current_count"
  lv_bms_data_a1/10 -> voltage_cell_3_bus/1  "voltage_cell_3"
  lv_bms_data_a1/11 -> soc_3_bus/1  "soc_3"
  lv_bms_data_a1/12 -> voltage_cell_4_bus/1  "voltage_cell_4"
  lv_bms_data_a1/13 -> soc_4_bus/1  "soc_4"
  lv_bms_data_a1/14 -> therm3_bus/1  "therm3"
  lv_bms_data_a1/15 -> voltage_cell_5_bus/1  "voltage_cell_5"
  lv_bms_data_a1/16 -> soc_5_bus/1  "soc_5"
  lv_bms_data_a1/17 -> therm4_bus/1  "therm4"
  lv_bms_data_a1/18 -> energy_count_bus/1  "energy_count"
  lv_bms_data_a1/19 -> voltage_cell_6_bus/1  "voltage_cell_6"
  lv_bms_data_a1/20 -> soc_6_bus/1  "soc_6"
  lv_bms_data_a1/21 -> therm5_bus/1  "therm5"
